simulink model "EXP3_simulink"  (R2015a)
settings: Solver=ode45  StartTime=0.0  StopTime=10.0  RelTol=1e-3
settings Model: Creator=meheli roy  LastModifiedBy=meheli roy

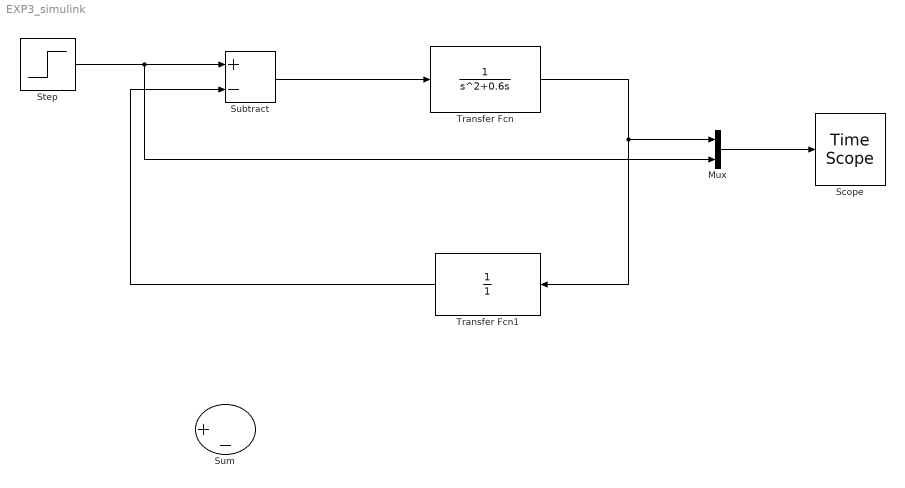
== system EXP3_simulink ==
  Mux : Mux  Inputs=2
  Scope : TimeScope
  Step : Step  Time=0  SampleTime=0
  Subtract : Sum  Inputs=+-
  Sum : Sum  Inputs=|+-
  Transfer Fcn : TransferFcn  Denominator=[1 0.6 0]
  Transfer Fcn1 : TransferFcn  Denominator=[1 ]
  wires:
  Transfer Fcn/1 -> Transfer Fcn1/1, Mux/1
  Subtract/1 -> Transfer Fcn/1
  Step/1 -> Mux/2, Subtract/1
  Transfer Fcn1/1 -> Subtract/2
  Mux/1 -> Scope/1
